simulink library "SLUGS_Library"  (Simulink 7.8)
settings: Solver=ode45  SolverMode=SingleTasking  StartTime=0.0  StopTime=10.0  RelTol=1e-3
values from neighbouring files (symbols this model uses):
  apSampleTime = 0.01    [mcuInit.m]
  derivativesConstant = 5    [mcuInit.m]
  latlong_WP = 1    [mcuInit.m]
  T = 0.01    [mcuInit.m]
  Xpoints = [0 0]    [mcuInit.m]
  Ypoints = [0 0]    [mcuInit.m]
  Zpoints = [0 0]    [mcuInit.m]
undefined symbols (not defined in the file or in its folder): bankCommandLimit, barAdjust, baroCutTemp, baroOffset, baroScale, barTGain1, barTGain2, barTMean1, barTMean2, baseHeight, baseTemp, daLimit, deLimit, DiscIntNeverNeededParam, drLimit, dtLimit, gaind, getGSLocation, getWP, GS_location, Init_onlyOnce, Init_Reset, IPStar, ISA_g, lapseRate, mass, maxAcc, MaxDwnPthStar, maxDynPressure, maxEta, Ndelay, param, pitAdjust, pitchCommandLimit, pitCutTemp, pitotOffset, pitotScale, pitTGain1, pitTGain2, pitTMean1, pitTMean2, polesd, pressureSensorCutoff, rollControlLimit, SampleT, setDiagnosticFloat, setDiagnosticShort, setLogFloat1, setLogFloat2, setNavLong, setNavNav, tanIntercept, Ts, u1, y1, yawDamperLimit, yo, zerosd
libraries: SLUGS_Library x90, simulink x37, dsPICdrivers x33, aerolibconvert2 x4, aerolibutil x1, aerolibobsolete x1
(part 5 of 7)

== system SLUGS_Library/Control Blocks/Lateral Channel/Roll Control [PID]/Trapezoidal Integrator ==
  x : Inport
  Reset : Inport  Port=2
  Constant : Constant  Value=1/3  OutDataTypeStr=single
  Constant1 : Constant  Value=4/3  OutDataTypeStr=single
  Constant2 : Constant  Value=T/2  OutDataTypeStr=single
  Constant3 : Constant  Value=1/3  OutDataTypeStr=single
  Constant5 : Constant  Value=0  OutDataTypeStr=single
  Integer Delay : Delay  DelayLength=1  InputProcessing=Inherited  SampleTime=T
  Integer Delay1 : Delay  InputProcessing=Inherited  SampleTime=T
  Integer Delay2 : Delay  DelayLength=1  InputProcessing=Inherited  SampleTime=T
  Product{,1..3} (4 alike) : Product  OutDataTypeStr=single  RndMeth=Zero
  "Protect NaNs " : Subsystem
  Protect NaNs1 : Subsystem
  Subtract : Sum  Inputs=3  OutDataTypeStr=single
  Subtract1 : Sum  Inputs=2  OutDataTypeStr=single
  Switch1 : Switch  Criteria=u2 > Threshold  Threshold=0.3  SampleTime=.01
  Int(x) : Outport
  wires:
  "Protect NaNs "/1(Out1) -> Product/1, Integer Delay/1, Integer Delay1/1
  Protect NaNs1/1(Out1) -> Int(x)/1, Integer Delay2/1
  Constant/1 -> Product/2
  Constant1/1 -> Product1/2
  Integer Delay/1 -> Product1/1
  Integer Delay1/1 -> Product2/1
  Constant3/1 -> Product2/2
  x/1 -> "Protect NaNs "/1(In1)
  Product/1 -> Subtract/1
  Product1/1 -> Subtract/2
  Product2/1 -> Subtract/3
  Constant2/1 -> Product3/1
  Subtract/1 -> Product3/2
  Subtract1/1 -> Switch1/3
  Integer Delay2/1 -> Subtract1/1
  Product3/1 -> Subtract1/2
  Constant5/1 -> Switch1/1
  Reset/1 -> Switch1/2
  Switch1/1 -> Protect NaNs1/1(In1)

== system SLUGS_Library/Control Blocks/Lateral Channel/Sideslip Compensation/Bank to Psi Dot ==
  phi_c : Inport
  U_m : Inport  Port=2
  Constant1 : Constant  Value=9.80665  OutDataTypeStr=single
  Divide : Product  Inputs=/*  OutDataTypeStr=single  SampleTime=apSampleTime
  Divide1 : Product  OutDataTypeStr=single  SampleTime=apSampleTime
  bank Limit : Saturate  UpperLimit=bankCommandLimit  LowerLimit=-bankCommandLimit
  dsPIC_tan : SLUGS_Library/dsPIC_tan
  negprotect : MATLAB Function  TreatAsAtomicUnit=on
  psi_dot_c : Outport
  wires:
  U_m/1 -> negprotect/1(val)
  Constant1/1 -> Divide/2
  Divide1/1 -> psi_dot_c/1
  dsPIC_tan/1 -> Divide1/1
  phi_c/1 -> bank Limit/1
  Divide/1 -> Divide1/2
  negprotect/1(zpVal) -> Divide/1
  bank Limit/1 -> dsPIC_tan/1

== system SLUGS_Library/Control Blocks/Lateral Channel/Sideslip Compensation/Low Pass ==
  a : Inport
  u : Inport  Port=2
  Compute Coef : Subsystem
  Detect Change : Subsystem
  Divide : Product  SampleTime=apSampleTime
  Divide1 : Product  SampleTime=apSampleTime
  IC : InitialCondition
  Integer Delay : Delay  DelayLength=1  InputProcessing=Inherited  SampleTime=apSampleTime
  Integer Delay1 : Delay  DelayLength=1  InputProcessing=Inherited  SampleTime=apSampleTime
  Subtract : Sum  SampleTime=apSampleTime
  y : Outport
  wires:
  Integer Delay1/1 -> Divide1/2
  u/1 -> Integer Delay/1
  IC/1 -> Compute Coef/Enable
  Subtract/1 -> Integer Delay1/1, y/1
  Divide1/1 -> Subtract/2
  Divide/1 -> Subtract/1
  Integer Delay/1 -> Divide/2
  Detect Change/1(change?) -> IC/1
  Compute Coef/2(c) -> Divide1/1
  Compute Coef/1(b) -> Divide/1
  a/1 -> Detect Change/1(Data), Compute Coef/1(a)

== system SLUGS_Library/Control Blocks/Lateral Channel/Sideslip Compensation/Protect NaNs2 ==
  In1 : Inport
  Integer Delay3 : Delay  DelayLength=1  InputProcessing=Inherited  SampleTime=T
  Relational Operator2 : RelationalOperator  Operator===  OutDataTypeStr=uint(8)
  Switch3 : Switch  Criteria=u2 > Threshold  Threshold=0.3  SampleTime=.01
  Out1 : Outport
  wires:
  Relational Operator2/1 -> Switch3/2
  In1/1 -> Switch3/1, Relational Operator2/1, Relational Operator2/2
  Switch3/1 -> Integer Delay3/1, Out1/1
  Integer Delay3/1 -> Switch3/3

== system SLUGS_Library/Control Blocks/Lateral Channel/Sideslip Compensation/psi_dot to Bank ==
  psi_dot_c : Inport
  U_m : Inport  Port=2
  Constant1 : Constant  Value=9.80665  OutDataTypeStr=single
  Divide : Product  Inputs=**/  SampleTime=apSampleTime
  dsPIC_atan : SLUGS_Library/dsPIC_atan
  phi_c : Outport
  wires:
  psi_dot_c/1 -> Divide/1
  U_m/1 -> Divide/2
  Constant1/1 -> Divide/3
  dsPIC_atan/1 -> phi_c/1
  Divide/1 -> dsPIC_atan/1

== system SLUGS_Library/Control Blocks/Lateral Channel/Yaw Damper [PID]/Trapezoidal Integrator ==
  x : Inport
  Reset : Inport  Port=2
  Constant : Constant  Value=1/3  OutDataTypeStr=single
  Constant1 : Constant  Value=4/3  OutDataTypeStr=single
  Constant2 : Constant  Value=T/2  OutDataTypeStr=single
  Constant3 : Constant  Value=1/3  OutDataTypeStr=single
  Constant5 : Constant  Value=0  OutDataTypeStr=single
  Integer Delay : Delay  DelayLength=1  InputProcessing=Inherited  SampleTime=T
  Integer Delay1 : Delay  InputProcessing=Inherited  SampleTime=T
  Integer Delay2 : Delay  DelayLength=1  InputProcessing=Inherited  SampleTime=T
  Product{,1..3} (4 alike) : Product  OutDataTypeStr=single  RndMeth=Zero
  "Protect NaNs " : Subsystem
  Protect NaNs1 : Subsystem
  Subtract : Sum  Inputs=3  OutDataTypeStr=single
  Subtract1 : Sum  Inputs=2  OutDataTypeStr=single
  Switch1 : Switch  Criteria=u2 > Threshold  Threshold=0.3  SampleTime=.01
  Int(x) : Outport
  wires:
  "Protect NaNs "/1(Out1) -> Product/1, Integer Delay/1, Integer Delay1/1
  Protect NaNs1/1(Out1) -> Int(x)/1, Integer Delay2/1
  Constant/1 -> Product/2
  Constant1/1 -> Product1/2
  Integer Delay/1 -> Product1/1
  Integer Delay1/1 -> Product2/1
  Constant3/1 -> Product2/2
  x/1 -> "Protect NaNs "/1(In1)
  Product/1 -> Subtract/1
  Product1/1 -> Subtract/2
  Product2/1 -> Subtract/3
  Constant2/1 -> Product3/1
  Subtract/1 -> Product3/2
  Subtract1/1 -> Switch1/3
  Integer Delay2/1 -> Subtract1/1
  Product3/1 -> Subtract1/2
  Constant5/1 -> Switch1/1
  Reset/1 -> Switch1/2
  Switch1/1 -> Protect NaNs1/1(In1)

== system SLUGS_Library/Control Blocks/Longitudinal Channel/Airspeed Hold [PID]/Trapezoidal Integrator ==
  x : Inport
  Reset : Inport  Port=2
  Constant : Constant  Value=1/3  OutDataTypeStr=single
  Constant1 : Constant  Value=4/3  OutDataTypeStr=single
  Constant2 : Constant  Value=T/2  OutDataTypeStr=single
  Constant3 : Constant  Value=1/3  OutDataTypeStr=single
  Constant5 : Constant  Value=0  OutDataTypeStr=single
  Integer Delay : Delay  DelayLength=1  InputProcessing=Inherited  SampleTime=T
  Integer Delay1 : Delay  InputProcessing=Inherited  SampleTime=T
  Integer Delay2 : Delay  DelayLength=1  InputProcessing=Inherited  SampleTime=T
  Product{,1..3} (4 alike) : Product  OutDataTypeStr=single  RndMeth=Zero
  "Protect NaNs " : Subsystem
  Protect NaNs1 : Subsystem
  Subtract : Sum  Inputs=3  OutDataTypeStr=single
  Subtract1 : Sum  Inputs=2  OutDataTypeStr=single
  Switch1 : Switch  Criteria=u2 > Threshold  Threshold=0.3  SampleTime=.01
  Int(x) : Outport
  wires:
  "Protect NaNs "/1(Out1) -> Product/1, Integer Delay/1, Integer Delay1/1
  Protect NaNs1/1(Out1) -> Int(x)/1, Integer Delay2/1
  Constant/1 -> Product/2
  Constant1/1 -> Product1/2
  Integer Delay/1 -> Product1/1
  Integer Delay1/1 -> Product2/1
  Constant3/1 -> Product2/2
  x/1 -> "Protect NaNs "/1(In1)
  Product/1 -> Subtract/1
  Product1/1 -> Subtract/2
  Product2/1 -> Subtract/3
  Constant2/1 -> Product3/1
  Subtract/1 -> Product3/2
  Subtract1/1 -> Switch1/3
  Integer Delay2/1 -> Subtract1/1
  Product3/1 -> Subtract1/2
  Constant5/1 -> Switch1/1
  Reset/1 -> Switch1/2
  Switch1/1 -> Protect NaNs1/1(In1)

== system SLUGS_Library/Control Blocks/Longitudinal Channel/Height Error to Pitch  Command [PI]/Trapezoidal Integrator ==
  x : Inport
  Reset : Inport  Port=2
  Constant : Constant  Value=1/3  OutDataTypeStr=single
  Constant1 : Constant  Value=4/3  OutDataTypeStr=single
  Constant2 : Constant  Value=T/2  OutDataTypeStr=single
  Constant3 : Constant  Value=1/3  OutDataTypeStr=single
  Constant5 : Constant  Value=0  OutDataTypeStr=single
  Integer Delay : Delay  DelayLength=1  InputProcessing=Inherited  SampleTime=T
  Integer Delay1 : Delay  InputProcessing=Inherited  SampleTime=T
  Integer Delay2 : Delay  DelayLength=1  InputProcessing=Inherited  SampleTime=T
  Product{,1..3} (4 alike) : Product  OutDataTypeStr=single  RndMeth=Zero
  Protect NaNs : Subsystem
  "Protect NaNs " : Subsystem
  Subtract : Sum  Inputs=3  OutDataTypeStr=single
  Subtract1 : Sum  Inputs=2  OutDataTypeStr=single
  Switch1 : Switch  Criteria=u2 > Threshold  Threshold=0.3  SampleTime=.01
  Int(x) : Outport
  wires:
  "Protect NaNs "/1(Out1) -> Integer Delay1/1, Integer Delay/1, Product/1
  Protect NaNs/1(Out1) -> Integer Delay2/1, Int(x)/1
  Switch1/1 -> Protect NaNs/1(In1)
  Reset/1 -> Switch1/2
  Constant5/1 -> Switch1/1
  Product3/1 -> Subtract1/2
  Integer Delay2/1 -> Subtract1/1
  Subtract1/1 -> Switch1/3
  Subtract/1 -> Product3/2
  Constant2/1 -> Product3/1
  Product2/1 -> Subtract/3
  Product1/1 -> Subtract/2
  Product/1 -> Subtract/1
  x/1 -> "Protect NaNs "/1(In1)
  Constant3/1 -> Product2/2
  Integer Delay1/1 -> Product2/1
  Integer Delay/1 -> Product1/1
  Constant1/1 -> Product1/2
  Constant/1 -> Product/2

== system SLUGS_Library/Control Blocks/Longitudinal Channel/Pitch To Elevator [PID]/Trapezoidal Integrator ==
  x : Inport
  Reset : Inport  Port=2
  Constant : Constant  Value=1/3  OutDataTypeStr=single
  Constant1 : Constant  Value=4/3  OutDataTypeStr=single
  Constant2 : Constant  Value=T/2  OutDataTypeStr=single
  Constant3 : Constant  Value=1/3  OutDataTypeStr=single
  Constant5 : Constant  Value=0  OutDataTypeStr=single
  Integer Delay : Delay  DelayLength=1  InputProcessing=Inherited  SampleTime=T
  Integer Delay1 : Delay  InputProcessing=Inherited  SampleTime=T
  Integer Delay2 : Delay  DelayLength=1  InputProcessing=Inherited  SampleTime=T
  Product{,1..3} (4 alike) : Product  OutDataTypeStr=single  RndMeth=Zero
  "Protect NaNs " : Subsystem
  Protect NaNs1 : Subsystem
  Subtract : Sum  Inputs=3  OutDataTypeStr=single
  Subtract1 : Sum  Inputs=2  OutDataTypeStr=single
  Switch1 : Switch  Criteria=u2 > Threshold  Threshold=0.3  SampleTime=.01
  Int(x) : Outport
  wires:
  "Protect NaNs "/1(Out1) -> Product/1, Integer Delay/1, Integer Delay1/1
  Protect NaNs1/1(Out1) -> Int(x)/1, Integer Delay2/1
  Constant/1 -> Product/2
  Constant1/1 -> Product1/2
  Integer Delay/1 -> Product1/1
  Integer Delay1/1 -> Product2/1
  Constant3/1 -> Product2/2
  x/1 -> "Protect NaNs "/1(In1)
  Product/1 -> Subtract/1
  Product1/1 -> Subtract/2
  Product2/1 -> Subtract/3
  Constant2/1 -> Product3/1
  Subtract/1 -> Product3/2
  Subtract1/1 -> Switch1/3
  Integer Delay2/1 -> Subtract1/1
  Product3/1 -> Subtract1/2
  Constant5/1 -> Switch1/1
  Reset/1 -> Switch1/2
  Switch1/1 -> Protect NaNs1/1(In1)

== system SLUGS_Library/Control Blocks/psi_dot_c Select logic/Bank to Psi Dot/Protect NaNs ==
  In1 : Inport
  Integer Delay3 : Delay  DelayLength=1  InputProcessing=Inherited  SampleTime=T
  Relational Operator2 : RelationalOperator  Operator===  OutDataTypeStr=uint(8)
  Switch3 : Switch  Criteria=u2 > Threshold  Threshold=0.3  SampleTime=.01
  Out1 : Outport
  wires:
  Integer Delay3/1 -> Switch3/3
  Switch3/1 -> Out1/1, Integer Delay3/1
  In1/1 -> Relational Operator2/2, Relational Operator2/1, Switch3/1
  Relational Operator2/1 -> Switch3/2

== system SLUGS_Library/Control Blocks/psi_dot_c Select logic/Bank to Psi Dot/Protect NaNs1 ==
  In1 : Inport
  Integer Delay3 : Delay  DelayLength=1  InputProcessing=Inherited  SampleTime=T
  Relational Operator2 : RelationalOperator  Operator===  OutDataTypeStr=uint(8)
  Switch3 : Switch  Criteria=u2 > Threshold  Threshold=0.3  SampleTime=.01
  Out1 : Outport
  wires:
  Relational Operator2/1 -> Switch3/2
  In1/1 -> Switch3/1, Relational Operator2/1, Relational Operator2/2
  Switch3/1 -> Integer Delay3/1, Out1/1
  Integer Delay3/1 -> Switch3/3

== system SLUGS_Library/InnerLoop/Longitudinal Channel/Air Density from Height/Subsystem ==
  u : Inport
  v : Inport  Port=2
  C Function Call : dsPICdrivers/OTHERS/C Function Call  Tag=dsPIC_dsPIC_CFunctionCall  FctUpdate=Output Function  fctName='myPow'  INPUT_SIZE=1  INPUT1=real32  INPUT2=real32  INPUT3=--  OUTPUT_SIZE=1  OUTPUT1=real32  SampleTime=-1  InputType=[ 7 7 ]  OutputType=[ 7 ]  FctDeclaration=extern real32_T myPow(real32_T u1, real32_T u2);  FctCall=%y1 = myPow(%u1, %u2);  OrderingInOutPopup=None  FctStart=None  FctStart_Name=Init_onlyOnce  FctStart_Declaration=inline extern void Init_onlyOnce();  FctStart_Call=Init_onlyOnce();  FctInit=None  FctInit_Name=Init_Reset  FctInit_Declaration=inline extern void Init_Reset();  FctInit_Call=Init_Reset();  PinDigitalInput=[]  PinDigitalOutput=[]  AnalogueInput=[]
  u^v : Outport
  wires:
  C Function Call/1 -> u^v/1
  u/1 -> C Function Call/1
  v/1 -> C Function Call/2

== system SLUGS_Library/InnerLoop/Longitudinal Channel/Airspeed Hold [PID]/Trapezoidal Integrator ==
  x : Inport
  Reset : Inport  Port=2
  Constant : Constant  Value=1/3  OutDataTypeStr=single
  Constant1 : Constant  Value=4/3  OutDataTypeStr=single
  Constant2 : Constant  Value=T/2  OutDataTypeStr=single
  Constant3 : Constant  Value=1/3  OutDataTypeStr=single
  Constant5 : Constant  Value=0  OutDataTypeStr=single
  Integer Delay : Delay  DelayLength=1  InputProcessing=Inherited  SampleTime=T
  Integer Delay1 : Delay  InputProcessing=Inherited  SampleTime=T
  Integer Delay2 : Delay  DelayLength=1  InputProcessing=Inherited  SampleTime=T
  Product{,1..3} (4 alike) : Product  OutDataTypeStr=single  RndMeth=Zero
  "Protect NaNs " : Subsystem
  Protect NaNs1 : Subsystem
  Subtract : Sum  Inputs=3  OutDataTypeStr=single
  Subtract1 : Sum  Inputs=2  OutDataTypeStr=single
  Switch1 : Switch  Criteria=u2 > Threshold  Threshold=0.3  SampleTime=.01
  Int(x) : Outport
  wires:
  Switch1/1 -> Protect NaNs1/1(In1)
  Reset/1 -> Switch1/2
  Constant5/1 -> Switch1/1
  Product3/1 -> Subtract1/2
  Integer Delay2/1 -> Subtract1/1
  Subtract1/1 -> Switch1/3
  Subtract/1 -> Product3/2
  Constant2/1 -> Product3/1
  Product2/1 -> Subtract/3
  Product1/1 -> Subtract/2
  Product/1 -> Subtract/1
  x/1 -> "Protect NaNs "/1(In1)
  Constant3/1 -> Product2/2
  Integer Delay1/1 -> Product2/1
  Integer Delay/1 -> Product1/1
  Constant1/1 -> Product1/2
  Constant/1 -> Product/2
  Protect NaNs1/1(Out1) -> Integer Delay2/1, Int(x)/1
  "Protect NaNs "/1(Out1) -> Integer Delay1/1, Integer Delay/1, Product/1

== system SLUGS_Library/InnerLoop/Longitudinal Channel/Compute Airspeed/Subsystem1 ==
  x : Inport
  C Function Call : dsPICdrivers/OTHERS/C Function Call  Tag=dsPIC_dsPIC_CFunctionCall  FctUpdate=Output Function  fctName='mySqrt'  INPUT_SIZE=1  INPUT1=real32  INPUT2=--  INPUT3=--  OUTPUT_SIZE=1  OUTPUT1=real32  SampleTime=-1  InputType=[ 7 ]  OutputType=[ 7 ]  FctDeclaration=extern real32_T mySqrt(real32_T u1);  FctCall=%y1 = mySqrt(%u1);  OrderingInOutPopup=None  FctStart=None  FctStart_Name=Init_onlyOnce  FctStart_Declaration=inline extern void Init_onlyOnce();  FctStart_Call=Init_onlyOnce();  FctInit=None  FctInit_Name=Init_Reset  FctInit_Declaration=inline extern void Init_Reset();  FctInit_Call=Init_Reset();  PinDigitalInput=[]  PinDigitalOutput=[]  AnalogueInput=[]
  negprotect : MATLAB Function  TreatAsAtomicUnit=on
  sqrt(x) : Outport
  wires:
  C Function Call/1 -> sqrt(x)/1
  negprotect/1(zpVal) -> C Function Call/1
  x/1 -> negprotect/1(val)

== system SLUGS_Library/InnerLoop/Longitudinal Channel/Height Error to Pitch  Command [PI]/Trapezoidal Integrator ==
  x : Inport
  Reset : Inport  Port=2
  Constant : Constant  Value=1/3  OutDataTypeStr=single
  Constant1 : Constant  Value=4/3  OutDataTypeStr=single
  Constant2 : Constant  Value=T/2  OutDataTypeStr=single
  Constant3 : Constant  Value=1/3  OutDataTypeStr=single
  Constant5 : Constant  Value=0  OutDataTypeStr=single
  Integer Delay : Delay  DelayLength=1  InputProcessing=Inherited  SampleTime=T
  Integer Delay1 : Delay  InputProcessing=Inherited  SampleTime=T
  Integer Delay2 : Delay  DelayLength=1  InputProcessing=Inherited  SampleTime=T
  Product{,1..3} (4 alike) : Product  OutDataTypeStr=single  RndMeth=Zero
  Protect NaNs : Subsystem
  "Protect NaNs " : Subsystem
  Subtract : Sum  Inputs=3  OutDataTypeStr=single
  Subtract1 : Sum  Inputs=2  OutDataTypeStr=single
  Switch1 : Switch  Criteria=u2 > Threshold  Threshold=0.3  SampleTime=.01
  Int(x) : Outport
  wires:
  Constant/1 -> Product/2
  Constant1/1 -> Product1/2
  Integer Delay/1 -> Product1/1
  Integer Delay1/1 -> Product2/1
  Constant3/1 -> Product2/2
  x/1 -> "Protect NaNs "/1(In1)
  Product/1 -> Subtract/1
  Product1/1 -> Subtract/2
  Product2/1 -> Subtract/3
  Constant2/1 -> Product3/1
  Subtract/1 -> Product3/2
  Subtract1/1 -> Switch1/3
  Integer Delay2/1 -> Subtract1/1
  Product3/1 -> Subtract1/2
  Constant5/1 -> Switch1/1
  Reset/1 -> Switch1/2
  Switch1/1 -> Protect NaNs/1(In1)
  Protect NaNs/1(Out1) -> Int(x)/1, Integer Delay2/1
  "Protect NaNs "/1(Out1) -> Product/1, Integer Delay/1, Integer Delay1/1

== system SLUGS_Library/InnerLoop/Longitudinal Channel/Pitch To Elevator [PID]/Trapezoidal Integrator ==
  x : Inport
  Reset : Inport  Port=2
  Constant : Constant  Value=1/3  OutDataTypeStr=single
  Constant1 : Constant  Value=4/3  OutDataTypeStr=single
  Constant2 : Constant  Value=T/2  OutDataTypeStr=single
  Constant3 : Constant  Value=1/3  OutDataTypeStr=single
  Constant5 : Constant  Value=0  OutDataTypeStr=single
  Integer Delay : Delay  DelayLength=1  InputProcessing=Inherited  SampleTime=T
  Integer Delay1 : Delay  InputProcessing=Inherited  SampleTime=T
  Integer Delay2 : Delay  DelayLength=1  InputProcessing=Inherited  SampleTime=T
  Product{,1..3} (4 alike) : Product  OutDataTypeStr=single  RndMeth=Zero
  "Protect NaNs " : Subsystem
  Protect NaNs1 : Subsystem
  Subtract : Sum  Inputs=3  OutDataTypeStr=single
  Subtract1 : Sum  Inputs=2  OutDataTypeStr=single
  Switch1 : Switch  Criteria=u2 > Threshold  Threshold=0.3  SampleTime=.01
  Int(x) : Outport
  wires:
  Switch1/1 -> Protect NaNs1/1(In1)
  Reset/1 -> Switch1/2
  Constant5/1 -> Switch1/1
  Product3/1 -> Subtract1/2
  Integer Delay2/1 -> Subtract1/1
  Subtract1/1 -> Switch1/3
  Subtract/1 -> Product3/2
  Constant2/1 -> Product3/1
  Product2/1 -> Subtract/3
  Product1/1 -> Subtract/2
  Product/1 -> Subtract/1
  x/1 -> "Protect NaNs "/1(In1)
  Constant3/1 -> Product2/2
  Integer Delay1/1 -> Product2/1
  Integer Delay/1 -> Product1/1
  Constant1/1 -> Product1/2
  Constant/1 -> Product/2
  Protect NaNs1/1(Out1) -> Integer Delay2/1, Int(x)/1
  "Protect NaNs "/1(Out1) -> Integer Delay1/1, Integer Delay/1, Product/1

== system SLUGS_Library/InnerLoop/Navigation/Compute WP Index/Compute Modified L1 ==
  WP1 : Inport
  T1 : Inport  Port=2
  WP2 : Inport  Port=3
  R : Inport  Port=4
  Enable : EnablePort  ShowOutputPort=on
  Compute T  in Frenet : Subsystem  AncestorBlock=SLUGS_Library/Navigation/Compute Frenet
  Get Circles : Subsystem
  Integer Delay1 : Delay  DelayLength=1  InputProcessing=Inherited
  Integer Delay2 : Delay  DelayLength=1  InputProcessing=Inherited
  To Workspace : ToWorkspace  VariableName=wpChange  SampleTime=-1  SaveFormat=Structure
  WP1_1 : InportShadow  Port=1
  get WP Coord from Index : Subsystem  AncestorBlock=SLUGS_Library/Navigation/get WP Coord from Index
  P : Outport
  wires:
  R/1 -> Get Circles/4(R)
  Enable/1 -> To Workspace/1
  Integer Delay1/1 -> Get Circles/1(T1)
  WP1_1/1 -> Get Circles/3("Wp_to ")
  Get Circles/1(P) -> P/1
  T1/1 -> Integer Delay1/1
  WP2/1 -> get WP Coord from Index/1(WP Idx)
  WP1/1 -> Compute T  in Frenet/1(Pos 1)
  Compute T  in Frenet/1(T) -> Get Circles/2(T2)
  Integer Delay2/1 -> Compute T  in Frenet/2(Pos 2)
  get WP Coord from Index/1(WP Coord) -> Integer Delay2/1

== system SLUGS_Library/InnerLoop/Navigation/Compute WP Index/Enabled Subsystem ==
  In1 : Inport
  Enable : EnablePort
  Out1 : Outport
  wires:
  In1/1 -> Out1/1

== system SLUGS_Library/InnerLoop/Navigation/Compute WP Index/Subsystem ==
  WP Fly : Inport
  Add1 : Sum  Inputs=2
  Hit  Crossing1 : HitCross  HitCrossingOffset=0.3  HitCrossingDirection=rising  SampleTime=apSampleTime
  Integer Delay1 : Delay  DelayLength=1  InitialCondition=0  InputProcessing=Inherited
  Just Enab : Outport
  wires:
  WP Fly/1 -> Hit  Crossing1/1
  Add1/1 -> Just Enab/1
  Hit  Crossing1/1 -> Integer Delay1/1, Add1/2
  Integer Delay1/1 -> Add1/1

== system SLUGS_Library/Navigation/Compute WP Index/Compute Modified L1/Compute T  in Frenet ==
  Pos 1 : Inport
  Pos 2 : Inport  Port=2
  Add : Sum  Inputs=-+
  Normalize Vector : SLUGS_Library/Navigation/Normalize Vector
  T : Outport
  wires:
  Normalize Vector/1 -> T/1
  Add/1 -> Normalize Vector/1
  Pos 2/1 -> Add/2
  Pos 1/1 -> Add/1

== system SLUGS_Library/Navigation/Compute WP Index/Compute Modified L1/Get Circles ==
  T1 : Inport
  T2 : Inport  Port=2
  "Wp_to " : Inport  Port=3
  R : Inport  Port=4
  Compute  Circles : MATLAB Function  TreatAsAtomicUnit=on
  Compute CCW Angle From 2 Vectors : Subsystem
  Compute delta Left Turn : Subsystem
  Constant5 : Constant  Value=pi
  Larger than 180? : RelationalOperator  OutDataTypeStr=boolean
  Logical Operator : Logic  Operator=NOT  AllPortsSameDT=off  OutDataTypeStr=boolean
  Merge4 : Merge
  Subsystem5 : SLUGS_Library/Subsystem5
  To Workspace : ToWorkspace  VariableName=O  SampleTime=-1  SaveFormat=Structure
  To Workspace1 : ToWorkspace  VariableName=P  SampleTime=-1  SaveFormat=Structure
  To Workspace2 : ToWorkspace  VariableName=Pch  SampleTime=-1  SaveFormat=Structure
  To Workspace3 : ToWorkspace  VariableName=PchB  SampleTime=-1  SaveFormat=Structure
  compute delta Right Turn : Subsystem
  P : Outport
  wires:
  T1/1 -> Compute  Circles/5(T1), Compute CCW Angle From 2 Vectors/1(U)
  Compute CCW Angle From 2 Vectors/1(CCW Ang) -> Compute delta Left Turn/1(gamma), compute delta Right Turn/1(gamma), Larger than 180?/1  "gamma"
  T2/1 -> Compute  Circles/6(T2), Compute CCW Angle From 2 Vectors/2(V)
  Merge4/1 -> Subsystem5/1
  compute delta Right Turn/1(delta) -> Merge4/1
  Compute delta Left Turn/1(delta) -> Merge4/2
  R/1 -> Compute  Circles/4(R)
  "Wp_to "/1 -> Compute  Circles/3(WP1)
  Compute  Circles/1(O) -> To Workspace/1
  Compute  Circles/2(P) -> P/1, To Workspace1/1
  Compute  Circles/3(Pch) -> To Workspace2/1
  Compute  Circles/4(PchB) -> To Workspace3/1
  Constant5/1 -> Larger than 180?/2
  Larger than 180?/1 -> compute delta Right Turn/Enable, Logical Operator/1
  Logical Operator/1 -> Compute delta Left Turn/Enable
  Subsystem5/1 -> Compute  Circles/1(sd)
  Subsystem5/2 -> Compute  Circles/2(cd)

== system SLUGS_Library/Navigation/Geod2LTP/ECEF2LTP (UEN)/From Body to Universal1 ==
  long : Inport
  lat : Inport  Port=2
  Mux : Mux  Inputs=2
  Reshape 9x1->3x1 : Reshape  OutputDimensionality=Customize  OutputDimensions=[3,3]
  Rotation Matrix from Long//Lat : Subsystem
      mask Type: Vector Transformation
      mask Description: Vector Transformation
      mask Display: disp('axis')
  DCM : Outport
  wires:
  Reshape 9x1->3x1/1 -> DCM/1
  Rotation Matrix from Long//Lat/1(DCM) -> Reshape 9x1->3x1/1
  Mux/1 -> Rotation Matrix from Long//Lat/1(long lat)
  long/1 -> Mux/1
  lat/1 -> Mux/2

== system SLUGS_Library/Navigation/Geod2LTP/Geod2ECEF1/eccentricity^2 ==
  " " : Product  OutDataTypeStr=single  SaturateOnIntegerOverflow=on  InputSameDT=on
  Re=equatorial radius1 : Constant  Value=Re  OutDataTypeStr=single
  Rp=polar radius : Constant  Value=Rp  OutDataTypeStr=single
  Sum5 : Sum  Inputs=|+-  SaturateOnIntegerOverflow=on  InputSameDT=on  OutDataTypeStr=Inherit: Same as first input
  const2 : Constant  OutDataTypeStr=single
  e^1 : Product  Inputs=*/  OutDataTypeStr=single  SaturateOnIntegerOverflow=on  InputSameDT=on
  e^2 : Outport
  wires:
  Sum5/1 -> e^2/1
  " "/1 -> Sum5/2
  e^1/1 -> " "/1, " "/2
  const2/1 -> Sum5/1
  Rp=polar radius/1 -> e^1/1
  Re=equatorial radius1/1 -> e^1/2

== system SLUGS_Library/Navigation/Navigation/Circle Navigation/Get SP Location ==
  GS LLA : Inport
  GS R_in : Inport  Port=2
  ISR Location : Inport  Port=3
  Demux : Demux  Outputs=3
  Geod2LTP : SLUGS_Library/Navigation/Geod2LTP
  Integer Delay1 : Delay  DelayLength=1  InputProcessing=Inherited
  Selector : Selector  InputPortWidth=3  IndexOptions=Index vector (dialog)  Indices=[3]  OutputSizes=1
  Zero out Z2 : MATLAB Function  TreatAsAtomicUnit=on
  Hc : Outport
  SP : Outport  Port=2
  wires:
  ISR Location/1 -> Demux/1
  GS R_in/1 -> Geod2LTP/2
  Demux/1 -> Geod2LTP/3
  Demux/2 -> Geod2LTP/4
  Demux/3 -> Geod2LTP/5
  GS LLA/1 -> Geod2LTP/1
  Geod2LTP/1 -> Zero out Z2/1(Pin), Selector/1
  Zero out Z2/1(P) -> SP/1
  Selector/1 -> Integer Delay1/1
  Integer Delay1/1 -> Hc/1

== system SLUGS_Library/Navigation/Navigation/Circle Navigation/Inside the Circle,  Keep Straight until  intersection ==
  ISR Loc : Inport
  R : Inport  Port=2
  Puav : Inport  Port=3
  Action Port : ActionPort
  Compute Head of Circle : MATLAB Function  TreatAsAtomicUnit=on
  RTB1 : Constant  OutDataTypeStr=uint8
  Subtract : Sum  Inputs=+-  OutDataTypeStr=single
  L2 Vec : Outport
  Mode : Outport  Port=2
  wires:
  Subtract/1 -> L2 Vec/1
  Puav/1 -> Subtract/2
  Compute Head of Circle/1(topCoord) -> Subtract/1
  ISR Loc/1 -> Compute Head of Circle/2(ISR)
  R/1 -> Compute Head of Circle/1(R)
  RTB1/1 -> Mode/1

== system SLUGS_Library/Navigation/Navigation/Circle Navigation/Intersection. Circular Navigation ==
  R : Inport
  L2 : Inport  Port=2
  d : Inport  Port=3
  ISR Loc : Inport  Port=4
  UAV m ISR : Inport  Port=5
  Vxyz : Inport  Port=6
  |Vg| : Inport  Port=7
  Puav : Inport  Port=8
  Action Port : ActionPort
  Compute Angle Between Vectors1 : SLUGS_Library/Compute Angle Between Vectors
  Compute Angle Between Vectors2 : SLUGS_Library/Compute Angle Between Vectors
  Embedded MATLAB Function : MATLAB Function  TreatAsAtomicUnit=on
  Product{,1..2,4..5,7} (6 alike) : Product  RndMeth=Zero
  Product3 : Product  Inputs=*/  RndMeth=Zero
  Product6 : Product  Inputs=*/  RndMeth=Zero
  RTB1 : Constant  Value=2  OutDataTypeStr=uint8
  Relational Operator : RelationalOperator  Operator=<=  OutDataTypeStr=boolean
  Subtract : Sum  Inputs=+-+
  Subtract1 : Sum  Inputs=2
  Subtract2 : Sum  Inputs=+-
  Subtract3 : Sum  Inputs=2
  Subtract5 : Sum  Inputs=+-
  Subtract6 : Sum  Inputs=-+
  Switch1 : Switch  Criteria=u2 > Threshold  Threshold=0.3  ZeroCross=off
  "d " : InportShadow  Port=3
  dsPIC_ABS : SLUGS_Library/dsPIC_ABS
  dsPIC_ABS1 : SLUGS_Library/dsPIC_ABS
  dsPIC_SQRT : SLUGS_Library/dsPIC_SQRT
  negprotect1 : MATLAB Function  TreatAsAtomicUnit=on
  negprotect2 : MATLAB Function  TreatAsAtomicUnit=on
  L2 Vec : Outport
  Mode : Outport  Port=2
  wires:
  Switch1/1 -> L2 Vec/1
  Puav/1 -> Subtract6/1, Subtract5/2
  Embedded MATLAB Function/2(P32) -> Subtract6/2
  Subtract6/1 -> Switch1/3, Compute Angle Between Vectors1/3
  Embedded MATLAB Function/1(P31) -> Subtract5/1
  Subtract5/1 -> Switch1/1, Compute Angle Between Vectors2/3
  Product5/1 -> Embedded MATLAB Function/1(hFact)
  dsPIC_SQRT/1 -> Product5/1  "h"
  RTB1/1 -> Mode/1
  Relational Operator/1 -> Switch1/2
  dsPIC_ABS/1 -> Relational Operator/2
  Compute Angle Between Vectors1/1 -> dsPIC_ABS/1
  dsPIC_ABS1/1 -> Relational Operator/1
  Compute Angle Between Vectors2/1 -> dsPIC_ABS1/1
  |Vg|/1 -> Compute Angle Between Vectors2/2, Compute Angle Between Vectors1/2
  Vxyz/1 -> Compute Angle Between Vectors2/1, Compute Angle Between Vectors1/1
  [UavMIsDbd] -> Product5/2
  [a] -> Product7/2
  Product6/1 -> [UavMIsDbd], Product7/1
  Product7/1 -> Subtract3/2
  UAV m ISR/1 -> Product6/1
  Subtract3/1 -> Embedded MATLAB Function/2(P2)  "P2"
  ISR Loc/1 -> Subtract3/1
  "d "/1 -> negprotect1/1(val)
  negprotect1/1(zpVal) -> Product6/2  "d"
  Subtract2/1 -> dsPIC_SQRT/1  "h"
  Product4/1 -> Subtract2/2  "a^2"
  Product3/1 -> [a], Product4/1, Product4/2  "a"
  Subtract1/1 -> negprotect2/1(val)
  negprotect2/1(zpVal) -> Product3/2  "2d"
  Subtract/1 -> Product3/1  "r^2 - L2^2 + d^2"
  Product2/1 -> Subtract/3
  Product1/1 -> Subtract/2
  Product/1 -> Subtract2/1, Subtract/1  "r^2"
  d/1 -> Subtract1/2, Subtract1/1, Product2/2, Product2/1
  L2/1 -> Product1/2, Product1/1
  R/1 -> Product/2, Product/1

== system SLUGS_Library/Navigation/Navigation/Circle Navigation/No intersection,  Navigate to ISR ==
  Puav : Inport
  ISR Loc : Inport  Port=2
  Action Port : ActionPort
  RTB1 : Constant  Value=0  OutDataTypeStr=uint8
  Subtract : Sum  Inputs=+-
  L2 Vec : Outport
  Mode : Outport  Port=2
  wires:
  RTB1/1 -> Mode/1
  Subtract/1 -> L2 Vec/1
  Puav/1 -> Subtract/2
  ISR Loc/1 -> Subtract/1

== system SLUGS_Library/Navigation/Navigation/L2+/Get Sin, Cos eta ==
  |V_g| : Inport
  L2_vec : Inport  Port=2
  Vxyz : Inport  Port=3
  "2D Dot Product " : Subsystem
  Compare To Zero : simulink/Logic and Bit Operations/Compare To Zero  relop===  OutDataTypeStr=uint8  ZeroCross=off
  Dead Zone : DeadZone  LowerValue=-0.1  UpperValue=0.1  SaturateOnIntegerOverflow=on
  Display : Display
  Display1 : Display
  Divide1 : Product  Inputs=/*
  Divide2 : Product  Inputs=*/
  Get  Groundspeed : Subsystem
  Get ZProd : Subsystem
  Product1 : Product  RndMeth=Zero
  Switch : Switch  Criteria=u2 > Threshold  Threshold=0.3  ZeroCross=off
  Switch2 : Switch  Criteria=u2 > Threshold  Threshold=0.3  ZeroCross=off
  cos(pi/2) : Constant  Value=0  OutDataTypeStr=single
  negprotect : MATLAB Function  TreatAsAtomicUnit=on
  sin(pi/2) : Constant  OutDataTypeStr=single
  sin(eta) : Outport
  cos(eta) : Outport  Port=2
  wires:
  Compare To Zero/1 -> Switch/2, Switch2/2
  Dead Zone/1 -> Compare To Zero/1
  L2_vec/1 -> Get ZProd/1(L2_vec), "2D Dot Product "/2(L2_vec), Get  Groundspeed/1(L2_vec)
  Vxyz/1 -> Get ZProd/2(Vxyz), "2D Dot Product "/1(Vxyz)
  Get  Groundspeed/1(|L2|) -> Product1/1
  |V_g|/1 -> Product1/2
  Product1/1 -> negprotect/1(val)
  "2D Dot Product "/1(2D _dot) -> Divide1/2
  sin(pi/2)/1 -> Switch/1
  Switch2/1 -> cos(eta)/1, Display1/1
  cos(pi/2)/1 -> Switch2/1
  Divide1/1 -> Switch2/3
  Get ZProd/1(Z_prod) -> Divide2/1
  Divide2/1 -> Switch/3
  Switch/1 -> sin(eta)/1, Display/1
  negprotect/1(zpVal) -> Dead Zone/1, Divide1/1, Divide2/2

== system SLUGS_Library/Navigation/Navigation/L2+/L2+ ==
  sin(eta) : Inport
  |V_g| : Inport  Port=2
  T* : Inport  Port=3
  Display3 : Display
  Divide : Product  Inputs=**/
  Gain : Gain  Gain=2  SampleTime=0.01
  negprotect : MATLAB Function  TreatAsAtomicUnit=on
  a_c : Outport
  wires:
  negprotect/1(zpVal) -> Divide/3
  sin(eta)/1 -> Divide/1
  Divide/1 -> Gain/1
  |V_g|/1 -> Divide/2
  Gain/1 -> a_c/1, Display3/1
  T*/1 -> negprotect/1(val)

== system SLUGS_Library/Navigation/Navigation/L2+/Subsystem ==
  a_c : Inport
  Bank  Limit Command : Saturate  UpperLimit=bankCommandLimit  LowerLimit=-bankCommandLimit  SampleTime=apSampleTime
  Constant : Constant  Value=ISA_g  OutDataTypeStr=single
  Product : Product  Inputs=*/  RndMeth=Zero
  To Workspace3 : ToWorkspace  VariableName=Phic  SampleTime=-1  SaveFormat=Array
  dsPIC_atan : SLUGS_Library/dsPIC_atan
  phi_c : Outport
  wires:
  a_c/1 -> Product/1
  Constant/1 -> Product/2
  Product/1 -> dsPIC_atan/1
  dsPIC_atan/1 -> Bank  Limit Command/1
  Bank  Limit Command/1 -> phi_c/1, To Workspace3/1

== system SLUGS_Library/Navigation/Navigation/L2+/if sin(eta) < 0 - maxAcc else                 maxAcc  ==
  sin(eta) : Inport
  Compare To Zero : simulink/Logic and Bit Operations/Compare To Zero  relop=<  OutDataTypeStr=uint8  ZeroCross=off
  Constant1 : Constant  Value=maxAcc  OutDataTypeStr=single
  Constant9 : Constant  Value=-maxAcc  OutDataTypeStr=single
  Switch1 : Switch  Criteria=u2 > Threshold  Threshold=0.3
  + - maxAcc : Outport
  wires:
  Compare To Zero/1 -> Switch1/2
  Constant9/1 -> Switch1/1
  Constant1/1 -> Switch1/3
  sin(eta)/1 -> Compare To Zero/1
  Switch1/1 -> + - maxAcc/1

== system SLUGS_Library/Navigation/Navigation/Normal WP  Navigation/Compute WP Switching Trigger ==
  ToWp : Inport
  T1 : Inport  Port=2
  N1 : Inport  Port=3
  LeadDistance : Inport  Port=4
  Puav : Inport  Port=5
  L2 : Inport  Port=6
  Add : Sum  Inputs=+-
  Add1 : Sum  Inputs=+-
  Add3 : Sum  Inputs=--
  Compute  Projection : Subsystem
  Constant1 : Constant  Value=0  OutDataTypeStr=single
  Constant3 : Constant  Value=MaxDwnPthStar  OutDataTypeStr=single
  Constant4 : Constant  Value=tanIntercept  OutDataTypeStr=single
  Divide : Product  Inputs=*/
  Divide1 : Product
  Product : Product  RndMeth=Zero
  Product1 : Product  RndMeth=Zero
  Product2 : Product  RndMeth=Zero
  "Puav " : InportShadow  Port=5
  Relational Operator : RelationalOperator  Operator=>  OutDataTypeStr=boolean
  Subtract : Sum  Inputs=+-  OutDataTypeStr=single
  Switch Distance Less than? : RelationalOperator  Operator=<  OutDataTypeStr=uint(8)  SampleTime=apSampleTime
  Switch1 : Switch  Criteria=u2 > Threshold  Threshold=0.3
  "T1 " : InportShadow  Port=2
  "WP1 " : InportShadow  Port=1
  dsPIC Dot Product : SLUGS_Library/dsPIC Dot Product
  dsPIC_ABS : SLUGS_Library/dsPIC_ABS
  dsPIC_SQRT : SLUGS_Library/dsPIC_SQRT
  max : SLUGS_Library/max
  max1 : SLUGS_Library/max
  min : SLUGS_Library/min
  Switch : Outport
  Dist2WP1 : Outport  Port=2
  L2Vec : Outport  Port=3
  wires:
  N1/1 -> dsPIC Dot Product/2
  Add3/1 -> L2Vec/1
  [Pwp1] -> Add3/2
  Product2/1 -> Add3/1
  "T1 "/1 -> Product2/2
  max/1 -> Product2/1
  Constant1/1 -> max/2
  Add1/1 -> max/1
  [Dwp1] -> Add1/1
  max1/1 -> Switch1/3
  Product1/1 -> Add/2
  [abs_e_N] -> Product1/1, Product1/2
  Product/1 -> Add/1
  [L2] -> Product/2, Product/1
  dsPIC_SQRT/1 -> max1/2
  Add/1 -> dsPIC_SQRT/1
  Switch1/1 -> Add1/2  "L2DownPath"
  [abs_e_N] -> Relational Operator/1
  [L2] -> Relational Operator/2
  Relational Operator/1 -> Switch1/2
  min/1 -> Switch1/1, max1/1  "minDownPath"
  Divide1/1 -> min/1
  Constant3/1 -> Divide1/2
  L2/1 -> [L2], Divide1/1
  Divide/1 -> min/2  "|e_N|/tanInt"
  Constant4/1 -> Divide/2
  dsPIC_ABS/1 -> [abs_e_N], Divide/1
  dsPIC Dot Product/1 -> dsPIC_ABS/1  "e_N"
  Subtract/1 -> [Pwp1], dsPIC Dot Product/1
  "WP1 "/1 -> Subtract/2
  "Puav "/1 -> Subtract/1
  Switch Distance Less than?/1 -> Switch/1
  T1/1 -> Compute  Projection/3(T)
  ToWp/1 -> Compute  Projection/2(ToWp)
  LeadDistance/1 -> Switch Distance Less than?/2
  Compute  Projection/1(D2wp1) -> [Dwp1], Dist2WP1/1, Switch Distance Less than?/1
  Puav/1 -> Compute  Projection/1(Pned)

== system SLUGS_Library/Navigation/Navigation/Normal WP  Navigation/Get Frenet ==
  GS LLA : Inport
  GS R_in : Inport  Port=2
  From WP : Inport  Port=3
  To WP : Inport  Port=4
  TurnLeadTime : Inport  Port=5
  |V_g| : Inport  Port=6
  Enable : EnablePort
  Compute Frenet : SLUGS_Library/Navigation/Compute Frenet
  Demux1 : Demux  Outputs=3
  GS LLA_1 : InportShadow  Port=1
  GS R_in_1 : InportShadow  Port=2
  Integer Delay1 : Delay  DelayLength=1  InitialCondition=1  InputProcessing=Inherited
  Product1 : Product  OutDataTypeStr=single  RndMeth=Zero
  To Workspace2 : ToWorkspace  VariableName=fromWP  SampleTime=-1  SaveFormat=Array
  To Workspace3 : ToWorkspace  VariableName=toWP  SampleTime=-1  SaveFormat=Array
  Zero out Z1 : MATLAB Function  TreatAsAtomicUnit=on
  Zero out Z2 : MATLAB Function  TreatAsAtomicUnit=on
  Zero out Z3 : MATLAB Function  TreatAsAtomicUnit=on
  get WP Coord from Index1 : SLUGS_Library/Navigation/get WP Coord from Index
  get WP Coord from Index2 : SLUGS_Library/Navigation/get WP Coord from Index
  H_c : Outport
  ToWp : Outport  Port=2
  T1 : Outport  Port=3
  N1 : Outport  Port=4
  TurnLeadDistance : Outport  Port=5
  wires:
  GS R_in_1/1 -> get WP Coord from Index2/3
  GS LLA_1/1 -> get WP Coord from Index2/2
  To WP/1 -> get WP Coord from Index2/1
  GS R_in/1 -> get WP Coord from Index1/3
  GS LLA/1 -> get WP Coord from Index1/2
  From WP/1 -> get WP Coord from Index1/1
  get WP Coord from Index2/1 -> Demux1/1, Zero out Z3/1(Pin), To Workspace3/1, Compute Frenet/2
  get WP Coord from Index1/1 -> To Workspace2/1, Compute Frenet/1
  Zero out Z1/1(P) -> N1/1
  Zero out Z2/1(P) -> T1/1
  Product1/1 -> TurnLeadDistance/1
  TurnLeadTime/1 -> Product1/1
  |V_g|/1 -> Product1/2
  Compute Frenet/1 -> Zero out Z2/1(Pin)
  Demux1/3 -> Integer Delay1/1
  Compute Frenet/2 -> Zero out Z1/1(Pin)
  Integer Delay1/1 -> H_c/1
  Zero out Z3/1(P) -> ToWp/1

== system SLUGS_Library/Navigation/Navigation/Normal WP  Navigation/On WP Enable ==
  L2 : Inport
  GS LLA : Inport  Port=2
  GS R_in : Inport  Port=3
  Enable : EnablePort
  Constant5 : Constant  Value=IPStar  OutDataTypeStr=single
  Product : Product  Inputs=3  RndMeth=Zero
  Subsystem : Subsystem
  Subtract : Sum  Inputs=+-
  P_i : Outport
  wires:
  Subsystem/1(WP0) -> Subtract/1
  Subsystem/2(T1) -> Product/2
  GS R_in/1 -> Subsystem/2(GS R_in)
  GS LLA/1 -> Subsystem/1(GS LLA)
  Subtract/1 -> P_i/1  "WP0 - L2*IP*T1"
  Product/1 -> Subtract/2
  L2/1 -> Product/1
  Constant5/1 -> Product/3

== system SLUGS_Library/Navigation/Navigation/RTB/Follow Mobile Navigation/Compute Mobile Location ==
  "Lat, Lon" : Inport
  GS LLA : Inport  Port=2
  GS R : Inport  Port=3
  Enable : EnablePort  StatesWhenEnabling=reset
  Demux4 : Demux  Outputs=2
  Geod2LTP : SLUGS_Library/Navigation/Geod2LTP
  No Height All in 2D : Constant  Value=0  OutDataTypeStr=single
  XYZ : Outport
  wires:
  GS LLA/1 -> Geod2LTP/1
  GS R/1 -> Geod2LTP/2
  No Height All in 2D/1 -> Geod2LTP/5
  Demux4/1 -> Geod2LTP/3
  Demux4/2 -> Geod2LTP/4
  "Lat, Lon"/1 -> Demux4/1
  Geod2LTP/1 -> XYZ/1

== system SLUGS_Library/Navigation/Navigation/RTB/Follow Mobile Navigation/Simple Predictor ==
  Base Point : Inport
  Discrete-Time Integrator : DiscreteIntegrator  InitialConditionSource=external  SampleTime=0.01  ICPrevOutput=DiscIntNeverNeededParam  ICPrevScaledInput=DiscIntNeverNeededParam
  Gain : Gain
  Gain1 : Gain  Gain=3
  Sum : Sum  Inputs=|+-
  Sum1 : Sum  Inputs=++|
  Predicted Bp : Outport
  wires:
  Sum1/1 -> Predicted Bp/1
  Base Point/1 -> Discrete-Time Integrator/2, Sum/1
  Gain1/1 -> Sum1/1
  Gain/1 -> Sum1/2, Sum/2
  Sum/1 -> Discrete-Time Integrator/1, Gain1/1
  Discrete-Time Integrator/1 -> Gain/1

== system SLUGS_Library/Navigation/Navigation/Recent Enable/Grab Upon Enable ==
  Enable : EnablePort
  Compute GS Location : Subsystem
  Constant : Constant  Value=GS_location  OutDataTypeStr=single
  Constant1 : Constant  Value=[0 36.988506 -122.055308]  OutDataTypeStr=single
  Data Type Conversion : DataTypeConversion  OutDataTypeStr=single
  Data Type Conversion1 : DataTypeConversion  OutDataTypeStr=single
  Demux : Demux  Outputs=[1 2]
  Environment Controller : simulink/Signal Routing/Environment Controller
  Get the GS Location [updateControlMCUState.c] : dsPICdrivers/OTHERS/C Function Call  Tag=dsPIC_dsPIC_CFunctionCall  FctUpdate=Output Function  fctName='getGSLocation'  INPUT_SIZE=1  INPUT1=--  INPUT2=--  INPUT3=--  OUTPUT_SIZE=3  OUTPUT1=real32  SampleTime=0.01  InputType=[ ]  OutputType=[ 7 ]  FctDeclaration=extern void getGSLocation(real32_T* y1);  FctCall=getGSLocation(*%y1);  OrderingInOutPopup=None  FctStart=None  FctStart_Name=Init_onlyOnce  FctStart_Declaration=inline extern void Init_onlyOnce();  FctStart_Call=Init_onlyOnce();  FctInit=None  FctInit_Name=Init_Reset  FctInit_Declaration=inline extern void Init_Reset();  FctInit_Call=Init_Reset();  PinDigitalInput=[]  PinDigitalOutput=[]  AnalogueInput=[]
  Terminator : Terminator
  Terminator1 : Terminator
  "GS, Lon, Lat" : Outport
  GS R_in : Outport  Port=2
  GS Altitude (m) : Outport  Port=3
  wires:
  Constant1/1 -> Terminator1/1
  Get the GS Location [updateControlMCUState.c]/1 -> Environment Controller/2
  Environment Controller/1 -> Demux/1, Compute GS Location/1(GS Location)
  Constant/1 -> Environment Controller/1
  Data Type Conversion1/1 -> GS R_in/1
  Data Type Conversion/1 -> "GS, Lon, Lat"/1
  Compute GS Location/1("Lon, Lat") -> Data Type Conversion/1
  Compute GS Location/2(R_in) -> Data Type Conversion1/1
  Demux/1 -> GS Altitude (m)/1
  Demux/2 -> Terminator/1

== system SLUGS_Library/Navigation/Navigation/Recent Enable/Subsystem ==
  WP Fly : Inport
  Data Type Conversion2 : DataTypeConversion  OutDataTypeStr=uint8  SampleTime=apSampleTime
  Detect Rising Edge : Subsystem
  Just Enab : Outport
  wires:
  Data Type Conversion2/1 -> Just Enab/1
  Detect Rising Edge/1(Out1) -> Data Type Conversion2/1
  WP Fly/1 -> Detect Rising Edge/1(In1)

== system SLUGS_Library/Sensor Blocks/Baro Alt/Baro Altimeter/Compute Barometric Height ==
  Base Height (m) : Inport
  Base Pressure (Pa) : Inport  Port=2
  Baro (Pa) : Inport  Port=3
  Constant2 : Constant  Value=baseTemp/(-LapseRate)  OutDataTypeStr=single
  Constant3 : Constant  Value=9.350253e-2  OutDataTypeStr=single
  Constant4 : Constant  Value=-1.888933e-1  OutDataTypeStr=single
  Constant5 : Constant  Value=2.180313e-5  OutDataTypeStr=single
  Divide : Product  Inputs=*/  OutDataTypeStr=single
  Divide{1..4} (4 alike) : Product  OutDataTypeStr=single
  Length Conversion : aerolibconvert2/Length Conversion  IU=ft  OU=m
  Sum1 : Sum  Inputs=|++  OutDataTypeStr=single
  Sum2 : Sum  Inputs=|+-  OutDataTypeStr=single
  Sum3 : Sum  Inputs=3  OutDataTypeStr=single
  "Altitude, m" : Outport
  wires:
  Length Conversion/1 -> Sum1/1
  Sum2/1 -> Divide/1
  Sum1/1 -> "Altitude, m"/1
  Divide3/1 -> Length Conversion/1
  Constant2/1 -> Divide3/2
  Sum3/1 -> Divide3/1
  Constant5/1 -> Sum3/3
  Divide2/1 -> Sum3/2
  Divide1/1 -> Sum3/1
  Constant4/1 -> Divide2/2
  Constant3/1 -> Divide1/2
  Divide4/1 -> Divide1/1  "x^2"
  Divide/1 -> Divide2/1, Divide4/1, Divide4/2  "x"
  Base Pressure (Pa)/1 -> Divide/2, Sum2/2
  Base Height (m)/1 -> Sum1/2
  Baro (Pa)/1 -> Sum2/1

== system SLUGS_Library/Sensor Blocks/Baro Alt/Baro Altimeter/Enabled Subsystem ==
  In1 : Inport
  Enable : EnablePort
  Out1 : Outport  InitialOutput=baseHeight
  wires:
  In1/1 -> Out1/1

== system SLUGS_Library/Sensor Blocks/Baro Alt/Baro Altimeter/GS Height ==
  Demux : Demux  Outputs=[1 2]
  Get the GS Location [updateSensorMCUState.c] : dsPICdrivers/OTHERS/C Function Call  Tag=dsPIC_dsPIC_CFunctionCall  FctUpdate=Output Function  fctName='getGSLocation'  INPUT_SIZE=1  INPUT1=--  INPUT2=--  INPUT3=--  OUTPUT_SIZE=3  OUTPUT1=real32  SampleTime=0.01  InputType=[ ]  OutputType=[ 7 ]  FctDeclaration=extern void getGSLocation(real32_T* y1);  FctCall=getGSLocation(*%y1);  OrderingInOutPopup=None  FctStart=None  FctStart_Name=Init_onlyOnce  FctStart_Declaration=inline extern void Init_onlyOnce();  FctStart_Call=Init_onlyOnce();  FctInit=None  FctInit_Name=Init_Reset  FctInit_Declaration=inline extern void Init_Reset();  FctInit_Call=Init_Reset();  PinDigitalInput=[]  PinDigitalOutput=[]  AnalogueInput=[]
  Terminator : Terminator
  GS Height : Outport
  wires:
  Get the GS Location [updateSensorMCUState.c]/1 -> Demux/1
  Demux/2 -> Terminator/1
  Demux/1 -> GS Height/1

== system SLUGS_Library/Sensor Blocks/Baro Alt/Baro Altimeter/Initial Baro Bias ==
  Baro (Pa) : Inport
  Enable : EnablePort
  Data Type Conversion : DataTypeConversion  OutDataTypeStr=double
  Data Type Conversion1 : DataTypeConversion  OutDataTypeStr=single
  Low Pass8 : Subsystem  mask(DiscretizedZeroPole){Zeros=[], Poles=[-3], Gain=3, AbsTol=auto, SampleTime=.01, method=tustin, Wc=1}
      mask prompts: Zeros "Zeros (enter in s-main:)"; Poles "Poles (enter in s-domain:)"; Gain "Gain (enter in s-domain:)"; AbsTol "Absolute tolerance:"; SampleTime "Sample time:"; Wc "Critical Frequency (Hz):"
      mask help: Continuous mask uses c2d to transform parameters onto the Discrete Zero-Pole block inside.
      mask init: same as SLUGS_Library/Singnal Routing & Conditioning/Filter
      mask StyleString: edit,edit,edit,edit,edit,popup(zoh|foh|tustin|prewarp|matched),edit
      mask CallbackString: |||||hidecrit|
      mask Display:
      | droots(zeross,poless,gainss)
      | text( 0.5, 1.0, method, 'verticalAlignment','top')
  "[80k - 120k]" : Saturate  UpperLimit=120000  LowerLimit=80000
  Baro (Gnd) : Outport
  wires:
  Baro (Pa)/1 -> Data Type Conversion/1
  Low Pass8/1(Out1) -> Data Type Conversion1/1
  Data Type Conversion/1 -> Low Pass8/1(In1)
  Data Type Conversion1/1 -> "[80k - 120k]"/1
  "[80k - 120k]"/1 -> Baro (Gnd)/1

== system SLUGS_Library/Sensor Blocks/Baro Alt/Baro Altimeter/Zero Out Height ==
  Base Height : Inport
  Computed Height : Inport  Port=2
  Enable : EnablePort
  Integer Delay : Delay  DelayLength=1  InitialCondition=0  InputProcessing=Inherited  SampleTime=.01
  Sum : Sum  Inputs=|+-  OutDataTypeStr=single
  Height Offset : Outport
  wires:
  Computed Height/1 -> Integer Delay/1
  Sum/1 -> Height Offset/1
  Integer Delay/1 -> Sum/2
  Base Height/1 -> Sum/1

== system SLUGS_Library/Sensor Blocks/Baro Alt/Temp Compensate Baro/Hi Temp Compensation ==
  Raw : Inport
  Temp Raw : Inport  Port=2
  Enable : EnablePort
  Add : Sum  OutDataTypeStr=single
  Constant : Constant  Value=barAdjust  OutDataTypeStr=single
  Divide1 : Product  OutDataTypeStr=single
  Mean Temperature for Calibration : Constant  Value=tempMean  OutDataTypeStr=single
  Sum1 : Sum  Inputs=|+-  OutDataTypeStr=single
  Sum2 : Sum  Inputs=|+-  OutDataTypeStr=single
  gains : Constant  Value=alpha  OutDataTypeStr=single
  Comp : Outport
  wires:
  Sum2/1 -> Add/2
  Add/1 -> Comp/1
  Constant/1 -> Add/1
  Divide1/1 -> Sum2/2
  gains/1 -> Divide1/1
  Sum1/1 -> Divide1/2
  Temp Raw/1 -> Sum1/1
  Raw/1 -> Sum2/1
  Mean Temperature for Calibration/1 -> Sum1/2

== system SLUGS_Library/Sensor Blocks/Baro Alt/Temp Compensate Baro/Lo Temp Compensation ==
  Raw : Inport
  Temp Raw : Inport  Port=2
  Enable : EnablePort
  Divide1 : Product  OutDataTypeStr=single
  Mean Temperature for Calibration : Constant  Value=tempMean  OutDataTypeStr=single
  Sum1 : Sum  Inputs=|+-  OutDataTypeStr=single
  Sum2 : Sum  Inputs=|+-  OutDataTypeStr=single
  gains : Constant  Value=alpha  OutDataTypeStr=single
  Comp : Outport
  wires:
  Mean Temperature for Calibration/1 -> Sum1/2
  Raw/1 -> Sum2/1
  Temp Raw/1 -> Sum1/1
  Sum1/1 -> Divide1/2
  gains/1 -> Divide1/1
  Divide1/1 -> Sum2/2
  Sum2/1 -> Comp/1

== system SLUGS_Library/Sensor Blocks/Pitot Sensor End/Temp Compensate Accel X1/Hi Temp Compensation2 ==
  Raw : Inport
  Temp Raw : Inport  Port=2
  Enable : EnablePort
  Divide1 : Product  OutDataTypeStr=single
  Mean Temperature for Calibration : Constant  Value=tempMean  OutDataTypeStr=single
  Sum1 : Sum  Inputs=|+-  OutDataTypeStr=single
  Sum2 : Sum  Inputs=|+-  OutDataTypeStr=single
  gains : Constant  Value=alpha  OutDataTypeStr=single
  Comp : Outport
  wires:
  Mean Temperature for Calibration/1 -> Sum1/2
  Raw/1 -> Sum2/1
  Temp Raw/1 -> Sum1/1
  Sum1/1 -> Divide1/2
  gains/1 -> Divide1/1
  Divide1/1 -> Sum2/2
  Sum2/1 -> Comp/1

== system SLUGS_Library/Sensor Blocks/Pitot Sensor End/Temp Compensate Accel X1/Lo Temp Compensation ==
  Raw : Inport
  Temp Raw : Inport  Port=2
  Enable : EnablePort
  Add : Sum  OutDataTypeStr=single
  Constant : Constant  Value=pitAdjust  OutDataTypeStr=single
  Divide1 : Product  OutDataTypeStr=single
  Mean Temperature for Calibration : Constant  Value=tempMean  OutDataTypeStr=single
  Sum1 : Sum  Inputs=|+-  OutDataTypeStr=single
  Sum2 : Sum  Inputs=|+-  OutDataTypeStr=single
  gains : Constant  Value=alpha  OutDataTypeStr=single
  Comp : Outport
  wires:
  Add/1 -> Comp/1
  Constant/1 -> Add/2
  Sum2/1 -> Add/1
  Divide1/1 -> Sum2/2
  gains/1 -> Divide1/1
  Sum1/1 -> Divide1/2
  Temp Raw/1 -> Sum1/1
  Raw/1 -> Sum2/1
  Mean Temperature for Calibration/1 -> Sum1/2

== system SLUGS_Library/Control Blocks/Control Blocks Examples/PI Controller w/Anti-Windup/Trapezoidal Integrator/Protect NaNs ==
  In1 : Inport
  Integer Delay3 : Delay  DelayLength=1  InputProcessing=Inherited  SampleTime=T
  Relational Operator2 : RelationalOperator  Operator===  OutDataTypeStr=uint(8)
  Switch3 : Switch  Criteria=u2 > Threshold  Threshold=0.3  SampleTime=.01
  Out1 : Outport
  wires:
  Integer Delay3/1 -> Switch3/3
  Switch3/1 -> Out1/1, Integer Delay3/1
  In1/1 -> Relational Operator2/2, Relational Operator2/1, Switch3/1
  Relational Operator2/1 -> Switch3/2

== system SLUGS_Library/Control Blocks/Control Blocks Examples/PI Controller w/Anti-Windup/Trapezoidal Integrator/Protect NaNs  ==
  In1 : Inport
  Integer Delay3 : Delay  DelayLength=1  InputProcessing=Inherited  SampleTime=T
  Relational Operator2 : RelationalOperator  Operator===  OutDataTypeStr=uint(8)
  Switch3 : Switch  Criteria=u2 > Threshold  Threshold=0.3  SampleTime=.01
  Out1 : Outport
  wires:
  Integer Delay3/1 -> Switch3/3
  Switch3/1 -> Out1/1, Integer Delay3/1
  In1/1 -> Relational Operator2/2, Relational Operator2/1, Switch3/1
  Relational Operator2/1 -> Switch3/2
